simulink model "kundur_two_area_system_closed_control"  (R2019a)
settings: Solver=VariableStepAuto  StartTime=0.0  StopTime=40  RelTol=1e-3
libraries: powerlib x43, powerlib_meascontrol x6, sps_avr x3, simulink x3
settings Model: Creator=Ram Baskar  LastModifiedBy=Ram Baskar

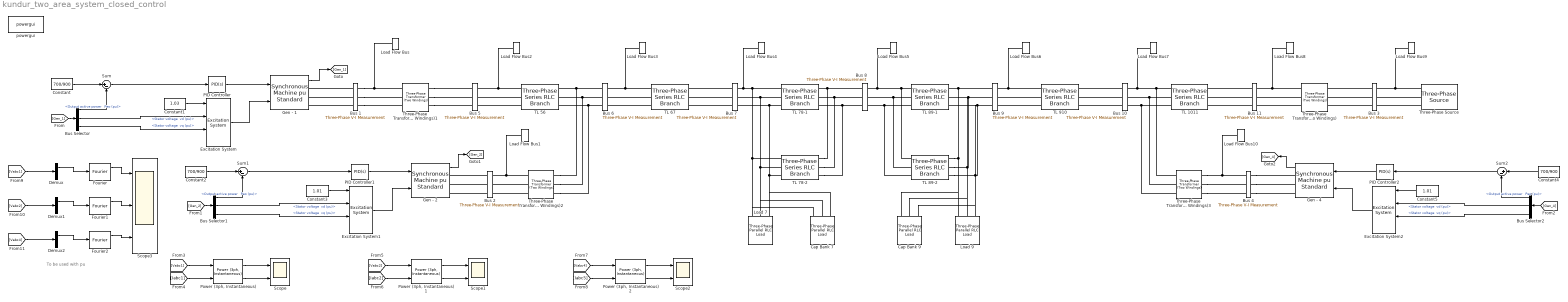
== system kundur_two_area_system_closed_control ==
  note: To be used with pu
  Bus Selector : BusSelector  OutputSignals="Output active power   Peo (pu),dq0 components.Stator voltage  vd (pu),dq0 components.Stator voltage  vq (pu)"
  Bus Selector1 : BusSelector  OutputSignals="Output active power   Peo (pu),dq0 components.Stator voltage  vd (pu),dq0 components.Stator voltage  vq (pu)"
  Bus Selector2 : BusSelector  OutputSignals="Output active power   Peo (pu),dq0 components.Stator voltage  vd (pu),dq0 components.Stator voltage  vq (pu)"
  Bus 1 : powerlib/Measurements/Three-Phase V-I Measurement  VoltageMeasurement=phase-to-ground  SetLabelV=on  LabelV=Vabc1  Vpu=off  VpuLL=off  CurrentMeasurement=yes  SetLabelI=on  LabelI=Iabc1  Ipu=off  Pbase=100e6  Vbase=20e3  OutputType=Complex  PhasorSimulation=off  PSBequivalent=0
      settings: SourceProductName=Simscape Electrical
  Bus 10 : powerlib/Measurements/Three-Phase V-I Measurement  VoltageMeasurement=phase-to-ground  SetLabelV=on  LabelV=Vabc10  Vpu=off  VpuLL=off  CurrentMeasurement=yes  SetLabelI=on  LabelI=Iabc10  Ipu=off  Pbase=100e6  Vbase=500e3  OutputType=Complex  PhasorSimulation=off  PSBequivalent=0
      settings: SourceProductName=Simscape Electrical
  Bus 11 : powerlib/Measurements/Three-Phase V-I Measurement  VoltageMeasurement=phase-to-ground  SetLabelV=on  LabelV=Vabc11  Vpu=off  VpuLL=off  CurrentMeasurement=yes  SetLabelI=on  LabelI=Iabc11  Ipu=off  Pbase=100e6  Vbase=500e3  OutputType=Complex  PhasorSimulation=off  PSBequivalent=0
      settings: SourceProductName=Simscape Electrical
  Bus 2 : powerlib/Measurements/Three-Phase V-I Measurement  VoltageMeasurement=phase-to-ground  SetLabelV=on  LabelV=Vabc2  Vpu=off  VpuLL=off  CurrentMeasurement=yes  SetLabelI=on  LabelI=Iabc2  Ipu=off  Pbase=100e6  Vbase=20e3  OutputType=Complex  PhasorSimulation=off  PSBequivalent=0
      settings: SourceProductName=Simscape Electrical
  Bus 3 : powerlib/Measurements/Three-Phase V-I Measurement  VoltageMeasurement=phase-to-ground  SetLabelV=on  LabelV=Vabc3  Vpu=off  VpuLL=off  CurrentMeasurement=yes  SetLabelI=on  LabelI=Iabc3  Ipu=off  Pbase=100e6  Vbase=500e3  OutputType=Complex  PhasorSimulation=off  PSBequivalent=0
      settings: SourceProductName=Simscape Electrical
  Bus 4 : powerlib/Measurements/Three-Phase V-I Measurement  VoltageMeasurement=phase-to-ground  SetLabelV=on  LabelV=Vabc4  Vpu=off  VpuLL=off  CurrentMeasurement=yes  SetLabelI=on  LabelI=Iabc4  Ipu=off  Pbase=100e6  Vbase=20e3  OutputType=Complex  PhasorSimulation=off  PSBequivalent=0
      settings: SourceProductName=Simscape Electrical
  Bus 5 : powerlib/Measurements/Three-Phase V-I Measurement  VoltageMeasurement=phase-to-ground  SetLabelV=on  LabelV=Vabc5  Vpu=off  VpuLL=off  CurrentMeasurement=yes  SetLabelI=on  LabelI=Iabc5  Ipu=off  Pbase=100e6  Vbase=500e3  OutputType=Complex  PhasorSimulation=off  PSBequivalent=0
      settings: SourceProductName=Simscape Electrical
  Bus 6 : powerlib/Measurements/Three-Phase V-I Measurement  VoltageMeasurement=phase-to-ground  SetLabelV=on  LabelV=Vabc6  Vpu=off  VpuLL=off  CurrentMeasurement=yes  SetLabelI=on  LabelI=Iabc6  Ipu=off  Pbase=100e6  Vbase=500e3  OutputType=Complex  PhasorSimulation=off  PSBequivalent=0
      settings: SourceProductName=Simscape Electrical
  Bus 7 : powerlib/Measurements/Three-Phase V-I Measurement  VoltageMeasurement=phase-to-ground  SetLabelV=on  LabelV=Vabc7  Vpu=off  VpuLL=off  CurrentMeasurement=yes  SetLabelI=on  LabelI=Iabc7  Ipu=off  Pbase=100e6  Vbase=500e3  OutputType=Complex  PhasorSimulation=off  PSBequivalent=0
      settings: SourceProductName=Simscape Electrical
  Bus 8 : powerlib/Measurements/Three-Phase V-I Measurement  VoltageMeasurement=phase-to-ground  SetLabelV=on  LabelV=Vabc8  Vpu=off  VpuLL=off  CurrentMeasurement=yes  SetLabelI=on  LabelI=Iabc8  Ipu=off  Pbase=100e6  Vbase=500e3  OutputType=Complex  PhasorSimulation=off  PSBequivalent=0
      settings: SourceProductName=Simscape Electrical
  Bus 9 : powerlib/Measurements/Three-Phase V-I Measurement  VoltageMeasurement=phase-to-ground  SetLabelV=on  LabelV=Vabc9  Vpu=off  VpuLL=off  CurrentMeasurement=yes  SetLabelI=on  LabelI=Iabc9  Ipu=off  Pbase=100e6  Vbase=500e3  OutputType=Complex  PhasorSimulation=off  PSBequivalent=0
      settings: SourceProductName=Simscape Electrical
  Cap Bank 7 : powerlib/Elements/Three-Phase Parallel RLC Load  LConnTagsString=A|B|C  Configuration=Y (grounded)  NominalVoltage=230e3*0.8958  Vabc=[1e3 1e3 1e3]  Vabcp=[1e3 1e3 1e3]  NominalFrequency=60  UnbalancedPower=off  ActivePower=0  InductivePower=0  CapacitivePower=200e6  Pabc=[10e3 9e3 11e3]  QLabc=[100 90 110]  QCabc=[100 90 110]  Pabcp=[10e3 9e3 11e3]  QLabcp=[100 90 110]  QCabcp=[100 90 110]  Measurements=Branch voltages and currents  LoadType=constant Z
      settings: SourceProductName=Simscape Electrical
  Cap Bank 9 : powerlib/Elements/Three-Phase Parallel RLC Load  LConnTagsString=A|B|C  Configuration=Y (grounded)  NominalVoltage=230e3*0.9667  Vabc=[1e3 1e3 1e3]  Vabcp=[1e3 1e3 1e3]  NominalFrequency=60  UnbalancedPower=off  ActivePower=0  InductivePower=0  CapacitivePower=350e6  Pabc=[10e3 9e3 11e3]  QLabc=[100 90 110]  QCabc=[100 90 110]  Pabcp=[10e3 9e3 11e3]  QLabcp=[100 90 110]  QCabcp=[100 90 110]  Measurements=Branch voltages and currents  LoadType=constant Z
      settings: SourceProductName=Simscape Electrical
  Constant : Constant  Value=700/900
  Constant1 : Constant  Value=1.03
  Constant2 : Constant  Value=700/900
  Constant3 : Constant  Value=1.01
  Constant4 : Constant  Value=700/900
  Constant5 : Constant  Value=1.01
  Demux : Demux  Outputs=3
  Demux1 : Demux  Outputs=3
  Demux2 : Demux  Outputs=3
  Excitation System : sps_avr/Excitation System  tr=0.05  reg=[ 20 0.055 ]  exc=[ 1 0 ]  tgr=[ 0 0 ]  damp=[ 0.125 1.8 ]  sat=[ 0, 0 ]  lim=[ -10 10 0 ]  v0=[0.97722 1.9731]
      settings: SourceProductName=Simscape Electrical  SourceProductBaseCode=PS
  Excitation System1 : sps_avr/Excitation System  tr=0.05  reg=[ 20 0.055 ]  exc=[ 1 0 ]  tgr=[ 0 0 ]  damp=[ 0.125 1.8 ]  sat=[ 0, 0 ]  lim=[ -10 10 0 ]  v0=[0.92899 2.0815]
      settings: SourceProductName=Simscape Electrical  SourceProductBaseCode=PS
  Excitation System2 : sps_avr/Excitation System  tr=0.05  reg=[ 20 0.055 ]  exc=[ 1 0 ]  tgr=[ 0 0 ]  damp=[ 0.125 1.8 ]  sat=[ 0, 0 ]  lim=[ -10 10 0 ]  v0=[0.99803 1.9844]
      settings: SourceProductName=Simscape Electrical  SourceProductBaseCode=PS
  Fourier : powerlib_meascontrol/Measurements/Fourier  Freq=60  n=1  InInit=[0, 0]  Ts=0
      settings: SourceProductName=Simscape Electrical
  Fourier1 : powerlib_meascontrol/Measurements/Fourier  Freq=60  n=1  InInit=[0, 0]  Ts=0
      settings: SourceProductName=Simscape Electrical
  Fourier2 : powerlib_meascontrol/Measurements/Fourier  Freq=60  n=1  InInit=[0, 0]  Ts=0
      settings: SourceProductName=Simscape Electrical
  Gen - 1 : powerlib/Machines/Synchronous Machine pu Standard  PresetModel=No  MechanicalLoad=Mechanical power Pm  ShowDetailedParameters=on  RotorType=Round  Units=per unit standard parameters  MeasurementBus=off  NominalParameters=[900e6 20e3 60]  Reactances1=[ 1.80 0.30 0.25 1.70 0.55 0.25 0.20 ]  Reactances2=[2.24 0.17 0.12 1.02 0.13 0.08]  dAxisTimeConstants=Open-circuit  qAxisTimeConstants=Open-circuit  TimeConstants1="[ 4.4849  0.0681  0.1  ]"  TimeConstants2=[ 8.0 0.03 0.40 0.05 ]  TimeConstants3="[  4.49  0.0681  0.0513  ]"  TimeConstants4=[ 8.0, 0.03, 0.3371, 0.0295 ]  TimeConstants5=[ 1.01, 0.053, 0.1 ]  TimeConstants6=[ 1.3201, 0.023, 1.0, 0.07 ]  TimeConstants7=[0.012 0.003 0.003]  TimeConstants8=[ 1.3201, 0.0231, 0.3371, 0.0295 ]  StatorResistance=0.0025  Mechanical=[6.50 0.02 1]  PolePairs=20  InitialConditions=[0 9.51314 0.823233 0.823233 0.823233 39.3744 -80.6256 159.374 1.97306]  SetSaturation=off  Saturation=[0.6404,0.7127,0.8441,0.9214,0.9956,1.082,1.19,1.316,1.457;0.7,0.7698,0.8872,0.9466,0.9969,1.046,1.1,1.151,1.201]  LoadFlowParameters=[1,0,0,0,0]  TsPowergui=0  TsBlock=-1  IterativeModel=Trapezoidal non iterative  IterativeDiscreteModel=Trapezoidal non iterative  BusType=PQ  Pref=700e6  Qref=185e6  Qmin=-inf  Qmax=inf  PLF=0  QLF=0
      settings: SourceProductName=Simscape Electrical
  Gen - 2 : powerlib/Machines/Synchronous Machine pu Standard  PresetModel=No  MechanicalLoad=Mechanical power Pm  ShowDetailedParameters=on  RotorType=Round  Units=per unit standard parameters  MeasurementBus=off  NominalParameters=[900e6 20e3 60]  Reactances1=[ 1.80 0.30 0.25 1.70 0.55 0.25 0.20 ]  Reactances2=[2.24 0.17 0.12 1.02 0.13 0.08]  dAxisTimeConstants=Open-circuit  qAxisTimeConstants=Open-circuit  TimeConstants1="[ 4.4849  0.0681  0.1  ]"  TimeConstants2=[ 8.0, 0.03, 0.40, 0.05 ]  TimeConstants3="[  4.49  0.0681  0.0513  ]"  TimeConstants4=[ 8.0, 0.03, 0.3371, 0.0295 ]  TimeConstants5=[ 1.01, 0.053, 0.1 ]  TimeConstants6=[ 1.3201, 0.023, 1.0, 0.07 ]  TimeConstants7=[0.012 0.003 0.003]  TimeConstants8=[ 1.3201, 0.0231, 0.3371, 0.0295 ]  StatorResistance=0.0025  Mechanical=[6.50 0.02 1]  PolePairs=20  InitialConditions=[0 -1.33613 0.88315 0.88315 0.88315 24.8293 -95.1707 144.829 2.08145]  SetSaturation=off  Saturation=[0.6404,0.7127,0.8441,0.9214,0.9956,1.082,1.19,1.316,1.457;0.7,0.7698,0.8872,0.9466,0.9969,1.046,1.1,1.151,1.201]  LoadFlowParameters=[1,0,0,0,0]  TsPowergui=0  TsBlock=-1  IterativeModel=Trapezoidal non iterative  IterativeDiscreteModel=Trapezoidal non iterative  BusType=PQ  Pref=700e6  Qref=235e6  Qmin=-inf  Qmax=inf  PLF=0  QLF=0
      settings: SourceProductName=Simscape Electrical
  Gen - 4 : powerlib/Machines/Synchronous Machine pu Standard  PresetModel=No  MechanicalLoad=Mechanical power Pm  ShowDetailedParameters=on  RotorType=Round  Units=per unit standard parameters  MeasurementBus=off  NominalParameters=[900e6 20e3 60]  Reactances1=[ 1.80 0.30 0.25 1.70 0.55 0.25 0.20 ]  Reactances2=[2.24 0.17 0.12 1.02 0.13 0.08]  dAxisTimeConstants=Open-circuit  qAxisTimeConstants=Open-circuit  TimeConstants1="[ 4.4849  0.0681  0.1  ]"  TimeConstants2=[ 8.0, 0.03, 0.40, 0.05 ]  TimeConstants3="[  4.49  0.0681  0.0513  ]"  TimeConstants4=[ 8.0, 0.03, 0.3371, 0.0295 ]  TimeConstants5=[ 1.01, 0.053, 0.1 ]  TimeConstants6=[ 1.3201, 0.023, 1.0, 0.07 ]  TimeConstants7=[0.012 0.003 0.003]  TimeConstants8=[ 1.3201, 0.0231, 0.3371, 0.0295 ]  StatorResistance=0.0025  Mechanical=[6.175 0.02 1]  PolePairs=20  InitialConditions=[0 -52.1606 0.811113 0.811113 0.811113 -22.0293 -142.029 97.9707 1.98442]  SetSaturation=off  Saturation=[0.6404,0.7127,0.8441,0.9214,0.9956,1.082,1.19,1.316,1.457;0.7,0.7698,0.8872,0.9466,0.9969,1.046,1.1,1.151,1.201]  LoadFlowParameters=[1,0,0,0,0]  TsPowergui=0  TsBlock=-1  IterativeModel=Trapezoidal non iterative  IterativeDiscreteModel=Trapezoidal non iterative  BusType=PQ  Pref=700e6  Qref=202e6  Qmin=-inf  Qmax=inf  PLF=0  QLF=0
      settings: SourceProductName=Simscape Electrical
  "Load 7 " : powerlib/Elements/Three-Phase Parallel RLC Load  LConnTagsString=A|B|C  Configuration=Y (grounded)  NominalVoltage=230e3*0.8958  Vabc=[1e3 1e3 1e3]  Vabcp=[1e3 1e3 1e3]  NominalFrequency=60  UnbalancedPower=off  ActivePower=967e6  InductivePower=100e6  CapacitivePower=0  Pabc=[10e3 9e3 11e3]  QLabc=[100 90 110]  QCabc=[100 90 110]  Pabcp=[10e3 9e3 11e3]  QLabcp=[100 90 110]  QCabcp=[100 90 110]  Measurements=Branch voltages and currents  LoadType=constant Z
      settings: SourceProductName=Simscape Electrical
  "Load 9 " : powerlib/Elements/Three-Phase Parallel RLC Load  LConnTagsString=A|B|C  Configuration=Y (grounded)  NominalVoltage=230e3*0.9667  Vabc=[1e3 1e3 1e3]  Vabcp=[1e3 1e3 1e3]  NominalFrequency=60  UnbalancedPower=off  ActivePower=1767e6  InductivePower=100e6  CapacitivePower=0  Pabc=[10e3 9e3 11e3]  QLabc=[100 90 110]  QCabc=[100 90 110]  Pabcp=[10e3 9e3 11e3]  QLabcp=[100 90 110]  QCabcp=[100 90 110]  Measurements=Branch voltages and currents  LoadType=constant Z
      settings: SourceProductName=Simscape Electrical
  Load Flow Bus : powerlib/Measurements/Load Flow Bus  LConnTagsString=a  Phases=single  Connectors=on one side  ID=BUS_1  Vbase=20e3  Vref=1  Vangle=0  VLF=0.9772  VLFb=1  VLFc=1  angleLF=54.18  angleLFb=0  angleLFc=0
      settings: SourceProductName=Simscape Electrical
  Load Flow Bus1 : powerlib/Measurements/Load Flow Bus  LConnTagsString=a  Phases=single  Connectors=on one side  ID=BUS_2  Vbase=20e3  Vref=1  Vangle=0  VLF=0.929  VLFb=1  VLFc=1  angleLF=43.39  angleLFb=0  angleLFc=0
      settings: SourceProductName=Simscape Electrical
  Load Flow Bus10 : powerlib/Measurements/Load Flow Bus  LConnTagsString=a  Phases=single  Connectors=on one side  ID=BUS_4  Vbase=20e3  Vref=1  Vangle=0  VLF=0.998  VLFb=1  VLFc=1  angleLF=-5.933  angleLFb=0  angleLFc=0
      settings: SourceProductName=Simscape Electrical
  Load Flow Bus2 : powerlib/Measurements/Load Flow Bus  LConnTagsString=a  Phases=single  Connectors=on one side  ID=BUS_5  Vbase=230e3  Vref=1  Vangle=0  VLF=0.9771  VLFb=1  VLFc=1  angleLF=54.16  angleLFb=0  angleLFc=0
      settings: SourceProductName=Simscape Electrical
  Load Flow Bus3 : powerlib/Measurements/Load Flow Bus  LConnTagsString=a  Phases=single  Connectors=on one side  ID=BUS_6  Vbase=230e3  Vref=1  Vangle=0  VLF=0.9289  VLFb=1  VLFc=1  angleLF=43.37  angleLFb=0  angleLFc=0
      settings: SourceProductName=Simscape Electrical
  Load Flow Bus4 : powerlib/Measurements/Load Flow Bus  LConnTagsString=a  Phases=single  Connectors=on one side  ID=BUS_7  Vbase=230e3  Vref=1  Vangle=0  VLF=0.8958  VLFb=1  VLFc=1  angleLF=34  angleLFb=0  angleLFc=0
      settings: SourceProductName=Simscape Electrical
  Load Flow Bus5 : powerlib/Measurements/Load Flow Bus  LConnTagsString=a  Phases=single  Connectors=on one side  ID=BUS_8  Vbase=230e3  Vref=1  Vangle=0  VLF=0.8557  VLFb=1  VLFc=1  angleLF=9.803  angleLFb=0  angleLFc=0
      settings: SourceProductName=Simscape Electrical
  Load Flow Bus6 : powerlib/Measurements/Load Flow Bus  LConnTagsString=a  Phases=single  Connectors=on one side  ID=BUS_9  Vbase=230e3  Vref=1  Vangle=0  VLF=0.9667  VLFb=1  VLFc=1  angleLF=-12.52  angleLFb=0  angleLFc=0
      settings: SourceProductName=Simscape Electrical
  Load Flow Bus7 : powerlib/Measurements/Load Flow Bus  LConnTagsString=a  Phases=single  Connectors=on one side  ID=BUS_10  Vbase=230e3  Vref=1  Vangle=0  VLF=0.9979  VLFb=1  VLFc=1  angleLF=-5.95  angleLFb=0  angleLFc=0
      settings: SourceProductName=Simscape Electrical
  Load Flow Bus8 : powerlib/Measurements/Load Flow Bus  LConnTagsString=a  Phases=single  Connectors=on one side  ID=BUS_11  Vbase=230e3  Vref=1  Vangle=0  VLF=1.03  VLFb=1  VLFc=1  angleLF=-0.01045  angleLFb=0  angleLFc=0
      settings: SourceProductName=Simscape Electrical
  Load Flow Bus9 : powerlib/Measurements/Load Flow Bus  LConnTagsString=a  Phases=single  Connectors=on one side  ID=BUS_3  Vbase=20e3  Vref=1.03  Vangle=0  VLF=1.03  VLFb=1  VLFc=1  angleLF=0  angleLFb=0  angleLFc=0
      settings: SourceProductName=Simscape Electrical
  PID Controller : simulink/Continuous/PID Controller  Controller=PID  Form=Parallel  TimeDomain=Continuous-time  SampleTime=-1  IntegratorMethod=Forward Euler  FilterMethod=Forward Euler  ControllerParametersSource=internal  P=1  I=2  D=0.2  UseFilter=on  N=100  TunerSelectOption=Transfer Function Based (PID Tuner App)  InitialConditionSource=internal  InitialConditionForIntegrator=0  InitialConditionForFilter=0  DifferentiatorICPrevScaledInput=0  ExternalReset=none  TrackingMode=off  Kt=1  LimitOutput=on  UpperSaturationLimit=0.99  LowerSaturationLimit=0.5  LinearizeAsGain=on  AntiWindupMode=none  Kb=1  POutMin=[]  POutMax=[]  IOutMin=[]  IOutMax=[]  DOutMin=[]  DOutMax=[]  NOutMin=[]  NOutMax=[]  SumOutMin=[]  SumOutMax=[]  SaturationOutMin=[]  SaturationOutMax=[]  PParamMin=[]  PParamMax=[]  IParamMin=[]  IParamMax=[]  DParamMin=[]  DParamMax=[]  NParamMin=[]  NParamMax=[]  KbParamMin=[]  KbParamMax=[]  KtParamMin=[]  KtParamMax=[]  KbOutMin=[]  KbOutMax=[]  KtOutMin=[]  KtOutMax=[]  IntegratorOutMin=[]  IntegratorOutMax=[]  FilterOutMin=[]  FilterOutMax=[]  SumI1OutMin=[]  SumI1OutMax=[]  SumI2OutMin=[]  SumI2OutMax=[]  SumI3OutMin=[]  SumI3OutMax=[]  SumI4OutMin=[]  SumI4OutMax=[]  SumDOutMin=[]  SumDOutMax=[]  DifferentiatorOutMin=[]  DifferentiatorOutMax=[]  FilterDiffOutCoefMin=[]  FilterDiffOutCoefMax=[]  ReciprocalOutMin=[]  ReciprocalOutMax=[]  SumDenOutMin=[]  SumDenOutMax=[]  SumNumOutMin=[]  SumNumOutMax=[]  DivideOutMin=[]  DivideOutMax=[]  IntegratorContinuousStateAttributes=''  IntegratorStateMustResolveToSignalObject=off  IntegratorRTWStateStorageClass=Auto  FilterContinuousStateAttributes=''  FilterStateMustResolveToSignalObject=off  FilterRTWStateStorageClass=Auto  ParallelPVariant=InternalParameters  IdealPVariant=Disabled  IVariant=InternalParameters  DVariant=InternalParameters  IntegratorVariant=Continuous  SatVariant=Enabled  AWVariant=Passthrough  PCopyVariant=Disabled  TRVariant=Disabled  FdbkBlocksVariant=Forward  IdealPFdbkVariant=Disabled  SatFdbkVariant=Disabled  DerivativeFilterVariant=ContFilter  NVariant=InternalParameters  NCopyVariant=Disabled  FilterICVariant=InternalICsFilter  IntegratorICVariant=InternalICs  ExternalResetVariant=Disabled  TRSumVariant=Passthrough  SumFdbkVariant=Disabled  SumVariant=Sum_PID
  PID Controller1 : simulink/Continuous/PID Controller  Controller=PID  Form=Parallel  TimeDomain=Continuous-time  SampleTime=-1  IntegratorMethod=Forward Euler  FilterMethod=Forward Euler  ControllerParametersSource=internal  P=1  I=2  D=0.2  UseFilter=on  N=100  TunerSelectOption=Transfer Function Based (PID Tuner App)  InitialConditionSource=internal  InitialConditionForIntegrator=0  InitialConditionForFilter=0  DifferentiatorICPrevScaledInput=0  ExternalReset=none  TrackingMode=off  Kt=1  LimitOutput=on  UpperSaturationLimit=0.99  LowerSaturationLimit=0.5  LinearizeAsGain=on  AntiWindupMode=none  Kb=1  POutMin=[]  POutMax=[]  IOutMin=[]  IOutMax=[]  DOutMin=[]  DOutMax=[]  NOutMin=[]  NOutMax=[]  SumOutMin=[]  SumOutMax=[]  SaturationOutMin=[]  SaturationOutMax=[]  PParamMin=[]  PParamMax=[]  IParamMin=[]  IParamMax=[]  DParamMin=[]  DParamMax=[]  NParamMin=[]  NParamMax=[]  KbParamMin=[]  KbParamMax=[]  KtParamMin=[]  KtParamMax=[]  KbOutMin=[]  KbOutMax=[]  KtOutMin=[]  KtOutMax=[]  IntegratorOutMin=[]  IntegratorOutMax=[]  FilterOutMin=[]  FilterOutMax=[]  SumI1OutMin=[]  SumI1OutMax=[]  SumI2OutMin=[]  SumI2OutMax=[]  SumI3OutMin=[]  SumI3OutMax=[]  SumI4OutMin=[]  SumI4OutMax=[]  SumDOutMin=[]  SumDOutMax=[]  DifferentiatorOutMin=[]  DifferentiatorOutMax=[]  FilterDiffOutCoefMin=[]  FilterDiffOutCoefMax=[]  ReciprocalOutMin=[]  ReciprocalOutMax=[]  SumDenOutMin=[]  SumDenOutMax=[]  SumNumOutMin=[]  SumNumOutMax=[]  DivideOutMin=[]  DivideOutMax=[]  IntegratorContinuousStateAttributes=''  IntegratorStateMustResolveToSignalObject=off  IntegratorRTWStateStorageClass=Auto  FilterContinuousStateAttributes=''  FilterStateMustResolveToSignalObject=off  FilterRTWStateStorageClass=Auto  ParallelPVariant=InternalParameters  IdealPVariant=Disabled  IVariant=InternalParameters  DVariant=InternalParameters  IntegratorVariant=Continuous  SatVariant=Enabled  AWVariant=Passthrough  PCopyVariant=Disabled  TRVariant=Disabled  FdbkBlocksVariant=Forward  IdealPFdbkVariant=Disabled  SatFdbkVariant=Disabled  DerivativeFilterVariant=ContFilter  NVariant=InternalParameters  NCopyVariant=Disabled  FilterICVariant=InternalICsFilter  IntegratorICVariant=InternalICs  ExternalResetVariant=Disabled  TRSumVariant=Passthrough  SumFdbkVariant=Disabled  SumVariant=Sum_PID
  PID Controller2 : simulink/Continuous/PID Controller  Controller=PID  Form=Parallel  TimeDomain=Continuous-time  SampleTime=-1  IntegratorMethod=Forward Euler  FilterMethod=Forward Euler  ControllerParametersSource=internal  P=1  I=2  D=0.2  UseFilter=on  N=100  TunerSelectOption=Transfer Function Based (PID Tuner App)  InitialConditionSource=internal  InitialConditionForIntegrator=0  InitialConditionForFilter=0  DifferentiatorICPrevScaledInput=0  ExternalReset=none  TrackingMode=off  Kt=1  LimitOutput=on  UpperSaturationLimit=0.99  LowerSaturationLimit=0.5  LinearizeAsGain=on  AntiWindupMode=none  Kb=1  POutMin=[]  POutMax=[]  IOutMin=[]  IOutMax=[]  DOutMin=[]  DOutMax=[]  NOutMin=[]  NOutMax=[]  SumOutMin=[]  SumOutMax=[]  SaturationOutMin=[]  SaturationOutMax=[]  PParamMin=[]  PParamMax=[]  IParamMin=[]  IParamMax=[]  DParamMin=[]  DParamMax=[]  NParamMin=[]  NParamMax=[]  KbParamMin=[]  KbParamMax=[]  KtParamMin=[]  KtParamMax=[]  KbOutMin=[]  KbOutMax=[]  KtOutMin=[]  KtOutMax=[]  IntegratorOutMin=[]  IntegratorOutMax=[]  FilterOutMin=[]  FilterOutMax=[]  SumI1OutMin=[]  SumI1OutMax=[]  SumI2OutMin=[]  SumI2OutMax=[]  SumI3OutMin=[]  SumI3OutMax=[]  SumI4OutMin=[]  SumI4OutMax=[]  SumDOutMin=[]  SumDOutMax=[]  DifferentiatorOutMin=[]  DifferentiatorOutMax=[]  FilterDiffOutCoefMin=[]  FilterDiffOutCoefMax=[]  ReciprocalOutMin=[]  ReciprocalOutMax=[]  SumDenOutMin=[]  SumDenOutMax=[]  SumNumOutMin=[]  SumNumOutMax=[]  DivideOutMin=[]  DivideOutMax=[]  IntegratorContinuousStateAttributes=''  IntegratorStateMustResolveToSignalObject=off  IntegratorRTWStateStorageClass=Auto  FilterContinuousStateAttributes=''  FilterStateMustResolveToSignalObject=off  FilterRTWStateStorageClass=Auto  ParallelPVariant=InternalParameters  IdealPVariant=Disabled  IVariant=InternalParameters  DVariant=InternalParameters  IntegratorVariant=Continuous  SatVariant=Enabled  AWVariant=Passthrough  PCopyVariant=Disabled  TRVariant=Disabled  FdbkBlocksVariant=Forward  IdealPFdbkVariant=Disabled  SatFdbkVariant=Disabled  DerivativeFilterVariant=ContFilter  NVariant=InternalParameters  NCopyVariant=Disabled  FilterICVariant=InternalICsFilter  IntegratorICVariant=InternalICs  ExternalResetVariant=Disabled  TRSumVariant=Passthrough  SumFdbkVariant=Disabled  SumVariant=Sum_PID
  "Power (3ph, Instantaneous)" : powerlib_meascontrol/Measurements/Power (3ph, Instantaneous)
      settings: SourceProductName=Simscape Electrical
  "Power (3ph, Instantaneous)1" : powerlib_meascontrol/Measurements/Power (3ph, Instantaneous)
      settings: SourceProductName=Simscape Electrical
  "Power (3ph, Instantaneous)2" : powerlib_meascontrol/Measurements/Power (3ph, Instantaneous)
      settings: SourceProductName=Simscape Electrical
  Scope : Scope  NumInputPorts=2
  Scope1 : Scope  NumInputPorts=2
  Scope2 : Scope  NumInputPorts=2
  Scope3 : Scope  NumInputPorts=3
  Sum : Sum  Inputs=|+-
  Sum1 : Sum  Inputs=|+-
  Sum2 : Sum  Inputs=|+-
  TL 1011 : powerlib/Elements/Three-Phase Series RLC Branch  LConnTagsString=A|B|C  RConnTagsString=A|B|C  BranchType=RL  Resistance=1.3225  Inductance=0.035080402  Capacitance=1e-6  Measurements=None
      settings: SourceProductName=Simscape Electrical
  TL 56 : powerlib/Elements/Three-Phase Series RLC Branch  LConnTagsString=A|B|C  RConnTagsString=A|B|C  BranchType=RL  Resistance=1.3225  Inductance=0.035080402  Capacitance=1e-6  Measurements=None
      settings: SourceProductName=Simscape Electrical
  "TL 67 " : powerlib/Elements/Three-Phase Series RLC Branch  LConnTagsString=A|B|C  RConnTagsString=A|B|C  BranchType=RL  Resistance=0.529  Inductance=1.403e-02  Capacitance=1e-6  Measurements=None
      settings: SourceProductName=Simscape Electrical
  TL 78-1 : powerlib/Elements/Three-Phase Series RLC Branch  LConnTagsString=A|B|C  RConnTagsString=A|B|C  BranchType=RL  Resistance=5.819  Inductance=1.5443e-01  Capacitance=1e-6  Measurements=None
      settings: SourceProductName=Simscape Electrical
  TL 78-2 : powerlib/Elements/Three-Phase Series RLC Branch  LConnTagsString=A|B|C  RConnTagsString=A|B|C  BranchType=RL  Resistance=5.819  Inductance=1.5443e-01  Capacitance=1e-6  Measurements=None
      settings: SourceProductName=Simscape Electrical
  TL 89-1 : powerlib/Elements/Three-Phase Series RLC Branch  LConnTagsString=A|B|C  RConnTagsString=A|B|C  BranchType=RL  Resistance=5.819  Inductance=1.5443e-01  Capacitance=1e-6  Measurements=None
      settings: SourceProductName=Simscape Electrical
  TL 89-2 : powerlib/Elements/Three-Phase Series RLC Branch  LConnTagsString=A|B|C  RConnTagsString=A|B|C  BranchType=RL  Resistance=5.819  Inductance=1.5443e-01  Capacitance=1e-6  Measurements=None
      settings: SourceProductName=Simscape Electrical
  "TL 910 " : powerlib/Elements/Three-Phase Series RLC Branch  LConnTagsString=A|B|C  RConnTagsString=A|B|C  BranchType=RL  Resistance=0.529  Inductance=1.403e-02  Capacitance=1e-6  Measurements=None
      settings: SourceProductName=Simscape Electrical
  Three-Phase Transformer (Two Windings){,1..3} (4 alike) : powerlib/Elements/Three-Phase Transformer (Two Windings)  Winding1Connection=Yg  Winding2Connection=Yg  CoreType=Three single-phase transformers  SetSaturation=off  Hysteresis=off  DataFile='hysteresis'  SetInitialFlux=off  Measurements=None  UNITS=pu  NominalPower=[ 900e6 , 60 ]  Winding1=[20e3 , 0 , 0.000198944 ]  Winding2=[ 230e3 , 0 , 0.000198944 ]  Rm=500  Lm=500  L0=0.5  Saturation=[ 0,0 ; 0.0024,1.2 ; 1.0,1.52 ]  InitialFluxes=[ 0.8 , -0.8 , 0.7 ]  BreakLoop=off  DiscreteSolver=Trapezoidal iterative  DataType=off  TransfoNumber=1
      settings: SourceProductName=Simscape Electrical
  Three-Phase Source : powerlib/Electrical Sources/Three-Phase Source  InternalConnection=Yg  VoltagePhases=off  Voltage=(20000)*1.03  PhaseAngle=0  Voltage_phases=[25e3 25e3 25e3]/sqrt(3)  PhaseAngles_phases=[0 -120 +120]  Frequency=60  NonIdealSource=off  SpecifyImpedance=off  Resistance=0.8929  Inductance=16.58e-3  ShortCircuitLevel=100e6  BaseVoltage=25e3  XRratio=7  BusType=swing  Pref=10e3  Qref=0  Prefabc=[10e3, 10e3, 10e3]  Qrefabc=[0, 0, 0]  Qmin=-inf  Qmax=inf
      settings: SourceProductName=Simscape Electrical
  powergui : powerlib/powergui  Priority=1  SimulationMode=Discrete  SampleTime=50e-6  frequency=60  Iterations=1000  frequencyindice=60  Pbase=100e6  ErrMax=0.0001  UnitsV=kV  UnitsW=MW  buscounter=0  FunctionMessages=off  echomessages=off  EnableUseOfTLC=off  CurrentSourceSwitches=off  DisableSnubberDevices=off  DisableRonSwitches=off  DisableVfSwitches=off  DisplayEquations=off  AutomaticDiscreteSolvers=on  SolverType=Tustin/Backward Euler (TBE)  Interpol=off  ExternalGateDelay=off  methode=off  Ts=100  x0status=blocks  SPID=on  SwTol=0  HookPort=off  NonlinearTolerance=0  nMaxIteration=15  ContinueOnMaxIteration=off  RestoreLinks=warning  ResistiveCurrentMeasurement=off  Frange=[0:2:500]  Ylog=off  Xlog=on  ShowGrid=off  save=off  variable=ZData  structure=0  ZoomFFT=off  StartTime=0.0  cycles=1  DisplayStyle=1  fundamental=60  FreqAxis=off  MaxFrequency=1000  frequencyindicesteady=1  RmsSteady=1  display=off
      settings: SourceProductName=Simscape Electrical
  wires:
  Sum/1 -> PID Controller/1
  Constant/1 -> Sum/1
  [Gen_1] -> Bus Selector/1
  Gen - 1/1 -> [Gen_1]
  PID Controller/1 -> Gen - 1/1
  Bus Selector/1 -> Sum/2  "<Output active power   Peo (pu)>"
  Constant1/1 -> Excitation System/1
  Bus Selector/2 -> Excitation System/2  "<Stator voltage  vd (pu)>"
  Bus Selector/3 -> Excitation System/3  "<Stator voltage  vq (pu)>"
  Excitation System/1 -> Gen - 1/2
  Sum1/1 -> PID Controller1/1
  Bus Selector1/2 -> Excitation System1/2  "<Stator voltage  vd (pu)>"
  Bus Selector1/3 -> Excitation System1/3  "<Stator voltage  vq (pu)>"
  Constant3/1 -> Excitation System1/1
  Bus Selector1/1 -> Sum1/2  "<Output active power   Peo (pu)>"
  PID Controller1/1 -> Gen - 2/1
  [Gen_2] -> Bus Selector1/1
  Excitation System1/1 -> Gen - 2/2
  Constant2/1 -> Sum1/1
  Sum2/1 -> PID Controller2/1
  Bus Selector2/2 -> Excitation System2/2  "<Stator voltage  vd (pu)>"
  Bus Selector2/3 -> Excitation System2/3  "<Stator voltage  vq (pu)>"
  Constant5/1 -> Excitation System2/1
  Bus Selector2/1 -> Sum2/2  "<Output active power   Peo (pu)>"
  PID Controller2/1 -> Gen - 4/1
  [Gen_4] -> Bus Selector2/1
  Excitation System2/1 -> Gen - 4/2
  Constant4/1 -> Sum2/1
  Gen - 2/1 -> [Gen_2]
  Gen - 4/1 -> [Gen_4]
  [Vabc1] -> "Power (3ph, Instantaneous)"/1
  [Iabc1] -> "Power (3ph, Instantaneous)"/2
  "Power (3ph, Instantaneous)"/1 -> Scope/1
  "Power (3ph, Instantaneous)"/2 -> Scope/2
  "Power (3ph, Instantaneous)1"/1 -> Scope1/1
  "Power (3ph, Instantaneous)1"/2 -> Scope1/2
  [Vabc2] -> "Power (3ph, Instantaneous)1"/1
  [Iabc2] -> "Power (3ph, Instantaneous)1"/2
  "Power (3ph, Instantaneous)2"/1 -> Scope2/1
  "Power (3ph, Instantaneous)2"/2 -> Scope2/2
  [Vabc4] -> "Power (3ph, Instantaneous)2"/1
  [Iabc5] -> "Power (3ph, Instantaneous)2"/2
  [Vabc1] -> Demux/1
  Demux/1 -> Fourier/1
  [Vabc2] -> Demux1/1
  Demux1/1 -> Fourier1/1
  [Vabc4] -> Demux2/1
  Demux2/1 -> Fourier2/1
  Fourier/1 -> Scope3/1
  Fourier1/1 -> Scope3/2
  Fourier2/1 -> Scope3/3
  connections:
  Bus 1/RConn1 -- Load Flow Bus/LConn1 -- Three-Phase Transformer (Two Windings)1/LConn1
  Bus 1/RConn2 -- Three-Phase Transformer (Two Windings)1/LConn2
  Bus 1/RConn3 -- Three-Phase Transformer (Two Windings)1/LConn3
  Bus 1/LConn2 -- Gen - 1/RConn2
  Bus 1/LConn3 -- Gen - 1/RConn3
  Bus 1/LConn1 -- Gen - 1/RConn1
  TL 56/LConn1 -- Load Flow Bus2/LConn1 -- Bus 5/RConn1
  TL 56/LConn2 -- Bus 5/RConn2
  TL 56/LConn3 -- Bus 5/RConn3
  Three-Phase Transformer (Two Windings)1/RConn2 -- Bus 5/LConn2
  Three-Phase Transformer (Two Windings)1/RConn3 -- Bus 5/LConn3
  Three-Phase Transformer (Two Windings)1/RConn1 -- Bus 5/LConn1
  Bus 6/LConn1 -- Three-Phase Transformer (Two Windings)2/RConn1 -- TL 56/RConn1
  Bus 6/LConn2 -- Three-Phase Transformer (Two Windings)2/RConn2 -- TL 56/RConn2
  Bus 6/LConn3 -- Three-Phase Transformer (Two Windings)2/RConn3 -- TL 56/RConn3
  "TL 67 "/LConn2 -- Bus 6/RConn2
  "TL 67 "/LConn3 -- Bus 6/RConn3
  "TL 67 "/LConn1 -- Load Flow Bus3/LConn1 -- Bus 6/RConn1
  Bus 7/LConn3 -- "TL 67 "/RConn3
  Bus 7/LConn1 -- "TL 67 "/RConn1
  Bus 7/LConn2 -- "TL 67 "/RConn2
  TL 78-1/LConn1 -- Cap Bank 7/LConn1 -- "Load 7 "/LConn1 -- TL 78-2/LConn1 -- Load Flow Bus4/LConn1 -- Bus 7/RConn1
  TL 78-1/LConn2 -- Cap Bank 7/LConn2 -- "Load 7 "/LConn2 -- TL 78-2/LConn2 -- Bus 7/RConn2
  TL 78-1/LConn3 -- Cap Bank 7/LConn3 -- "Load 7 "/LConn3 -- TL 78-2/LConn3 -- Bus 7/RConn3
  Bus 8/LConn1 -- TL 78-2/RConn1 -- TL 78-1/RConn1
  Bus 8/LConn2 -- TL 78-2/RConn2 -- TL 78-1/RConn2
  Bus 8/LConn3 -- TL 78-2/RConn3 -- TL 78-1/RConn3
  TL 89-1/LConn1 -- TL 89-2/LConn1 -- Load Flow Bus5/LConn1 -- Bus 8/RConn1
  TL 89-1/LConn2 -- TL 89-2/LConn2 -- Bus 8/RConn2
  TL 89-1/LConn3 -- TL 89-2/LConn3 -- Bus 8/RConn3
  Bus 9/LConn1 -- TL 89-1/RConn1 -- Cap Bank 9/LConn1 -- "Load 9 "/LConn1 -- TL 89-2/RConn1
  Bus 9/LConn2 -- Cap Bank 9/LConn2 -- "Load 9 "/LConn2 -- TL 89-2/RConn2 -- TL 89-1/RConn2
  Bus 9/LConn3 -- Cap Bank 9/LConn3 -- "Load 9 "/LConn3 -- TL 89-2/RConn3 -- TL 89-1/RConn3
  "TL 910 "/LConn1 -- Load Flow Bus6/LConn1 -- Bus 9/RConn1
  "TL 910 "/LConn2 -- Bus 9/RConn2
  "TL 910 "/LConn3 -- Bus 9/RConn3
  Bus 10/LConn1 -- "TL 910 "/RConn1
  Bus 10/LConn2 -- "TL 910 "/RConn2
  Bus 10/LConn3 -- "TL 910 "/RConn3
  TL 1011/LConn1 -- Three-Phase Transformer (Two Windings)3/RConn1 -- Load Flow Bus7/LConn1 -- Bus 10/RConn1
  TL 1011/LConn2 -- Three-Phase Transformer (Two Windings)3/RConn2 -- Bus 10/RConn2
  TL 1011/LConn3 -- Three-Phase Transformer (Two Windings)3/RConn3 -- Bus 10/RConn3
  Bus 11/LConn1 -- TL 1011/RConn1
  Bus 11/LConn2 -- TL 1011/RConn2
  Bus 11/LConn3 -- TL 1011/RConn3
  Three-Phase Transformer (Two Windings)/RConn1 -- Load Flow Bus8/LConn1 -- Bus 11/RConn1
  Three-Phase Transformer (Two Windings)/RConn2 -- Bus 11/RConn2
  Three-Phase Transformer (Two Windings)/RConn3 -- Bus 11/RConn3
  Bus 3/LConn1 -- Three-Phase Transformer (Two Windings)/LConn1
  Bus 3/LConn2 -- Three-Phase Transformer (Two Windings)/LConn2
  Bus 3/LConn3 -- Three-Phase Transformer (Two Windings)/LConn3
  Three-Phase Source/RConn1 -- Load Flow Bus9/LConn1 -- Bus 3/RConn1
  Three-Phase Source/RConn2 -- Bus 3/RConn2
  Three-Phase Source/RConn3 -- Bus 3/RConn3
  Bus 2/LConn2 -- Gen - 2/RConn2
  Bus 2/LConn1 -- Gen - 2/RConn1
  Bus 2/LConn3 -- Gen - 2/RConn3
  Three-Phase Transformer (Two Windings)2/LConn1 -- Load Flow Bus1/LConn1 -- Bus 2/RConn1
  Three-Phase Transformer (Two Windings)2/LConn2 -- Bus 2/RConn2
  Three-Phase Transformer (Two Windings)2/LConn3 -- Bus 2/RConn3
  Bus 4/LConn1 -- Gen - 4/RConn1
  Bus 4/LConn3 -- Gen - 4/RConn3
  Bus 4/LConn2 -- Gen - 4/RConn2
  Three-Phase Transformer (Two Windings)3/LConn1 -- Load Flow Bus10/LConn1 -- Bus 4/RConn1
  Three-Phase Transformer (Two Windings)3/LConn3 -- Bus 4/RConn3
  Three-Phase Transformer (Two Windings)3/LConn2 -- Bus 4/RConn2
